simulink model "interpolation_nD_TestGen65"  (R2017b)
settings: Solver=FixedStepDiscrete  StartTime=0.0  StopTime=10.0  RelTol=1e-3
settings Model: Creator=ktrinh  LastModifiedBy=ktrinh
settings DebuggingCC: ParameterOverflowMsg=none

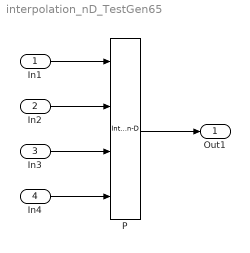
== system interpolation_nD_TestGen65 ==
  In1 : Inport  OutMin=0  OutMax=2  OutDataTypeStr=Bus: kfBus  PortDimensions=1  BusOutputAsStruct=on
  In2 : Inport  Port=2  OutMin=0  OutMax=5  OutDataTypeStr=Bus: kfBus  BusOutputAsStruct=on
  In3 : Inport  Port=3  OutMin=0  OutMax=3  OutDataTypeStr=Bus: kfBus  BusOutputAsStruct=on
  In4 : Inport  Port=4  OutMin=0  OutMax=2
  P : Interpolation_n-D  InitFcn=|  NumberOfTableDimensions=4  Table=reshape(repmat([4 5 6 7 8;16 19 20 21 22;10 18 23 24 25],2,2),[2,5,3,2])  RequireIndexFractionAsBus=on  ValidIndexMayReachLast=on  NumSelectionDims=1  InternalRulePriority=Speed  SaturateOnIntegerOverflow=on
      | elems(1) = Simulink.BusElement;
      | elems(1).Name = 'Index';
      | elems(1).DataType = 'int8';
      | elems(2) = Simulink.BusElement;
      | elems(2).Name = 'Fraction';
      | elems(2).DataType = 'double';
      | kfBus = Simulink.Bus;
      | kfBus.Elements = elems;
      | clear elems;
      | assignin('base', 'kfBus', kfBus);
  Out1 : Outport
  wires:
  In1/1 -> P/1
  In2/1 -> P/2
  In3/1 -> P/3
  In4/1 -> P/4
  P/1 -> Out1/1
